simulink model "Pilot"  (R2023b)
settings: Solver=FixedStepAuto  StartTime=0.0  StopTime=inf  FixedStep=sample_time  RelTol=1e-3
model workspace (MAT data in the model file):
  SL_ROS_VariableLengthArrays_MaxSizes.CommonInfo.ArrayTruncateAction = 'EmitWarning'
  SL_ROS_VariableLengthArrays_MaxSizes.MsgTypeMap = containers.Map
  SL_ROS_VariableLengthArrays_MaxSizes.MsgTypeMap.serialization.keys = {'sensor_msgs/Image'}
  SL_ROS_VariableLengthArrays_MaxSizes.MsgTypeMap.serialization.values{1}(1).PropertyName = 'data'
  SL_ROS_VariableLengthArrays_MaxSizes.MsgTypeMap.serialization.values{1}(1).DataType = 'uint8'
  SL_ROS_VariableLengthArrays_MaxSizes.MsgTypeMap.serialization.values{1}(1).MaxLength = 921600
  SL_ROS_VariableLengthArrays_MaxSizes.MsgTypeMap.serialization.values{1}(2).PropertyName = 'encoding'
  SL_ROS_VariableLengthArrays_MaxSizes.MsgTypeMap.serialization.values{1}(2).DataType = 'uint8'
  SL_ROS_VariableLengthArrays_MaxSizes.MsgTypeMap.serialization.values{1}(2).MaxLength = 128
  SL_ROS_VariableLengthArrays_MaxSizes.MsgTypeMap.serialization.uniformity = 0
  SL_ROS_VariableLengthArrays_MaxSizes.MsgTypeMap.serialization.keyType = 'char'
  SL_ROS_VariableLengthArrays_MaxSizes.MsgTypeMap.serialization.valueType = 'any'
  sample_time = 0.1
undefined symbols (not defined in the file or in its folder): duration, vel
libraries: ros2lib x2, vrlib x1, simulink_extras x1
settings Model: Creator=rcasado  LastModifiedBy=Rafa
settings SolverCC: AlgebraicLoopSolver=TrustRegion
settings DataIOCC: ReturnWorkspaceOutputs=off
settings OptimizationCC: EnhancedBackFolding=on  PassReuseOutputArgsAs=Individual arguments  ZeroExternalMemoryAtStartup=off  ZeroInternalMemoryAtStartup=off  MaxStackSize=64  OptimizeBlockOrder=speed  DifferentSizesBufferReuse=on  OptimizationCustomize=off  EfficientTunableParamExpr=on
settings DebuggingCC: ParameterTunabilityLossMsg=error  UnconnectedInputMsg=warning  UnconnectedOutputMsg=warning  UnconnectedLineMsg=warning  BusObjectLabelMismatch=none  PregeneratedLibrarySubsystemCodeDiagnostic=none  ArithmeticOperatorsInVariantConditions=warning
settings HardwareCC: ProdBitPerPointer=32  ProdBitPerSizeT=32  ProdBitPerPtrDiffT=32  ProdLargestAtomicFloat=None  ProdIntDivRoundTo=Undefined  ProdEndianess=Unspecified  ProdWordSize=32  ProdHWDeviceType=Generic->Unspecified (assume 32-bit Generic)
settings ModelReferenceCC: EnableRefExpFcnMdlSchedulingChecks=on
settings SFSimCC: SimUseLocalCustomCode=off  CustomCodeUndefinedFunction=UseInterfaceOnly  SimTargetLang=C++
settings RTWCC: Description=Embedded Coder  SystemTargetFile=ert.tlc  HardwareBoard=Robot Operating System (ROS)  TLCOptions="-aInlineSetEventsForThisBaseRateFcn=TLC_FALSE -aSuppressMultiTaskScheduler=TLC_FALSE  -aRateBasedStepFcn=0"  TemplateMakefile=ert_default_tmf  GenerateReport=on  RTWUseLocalCustomCode=off  Toolchain=Catkin  IncludeHyperlinkInReport=on  LaunchReport=on  TargetLang=C++  GenerateTraceInfo=on  GenerateTraceReport=on  GenerateTraceReportSl=on  GenerateTraceReportSf=on  GenerateTraceReportEml=on  DLArmComputeVersion=19.05
settings CodeAppCC: ForceParamTrailComments=on  IgnoreCustomStorageClasses=off  OperatorAnnotations=on  SimulinkDataObjDesc=on  SFDataObjDesc=on  InsertBlockDesc=on

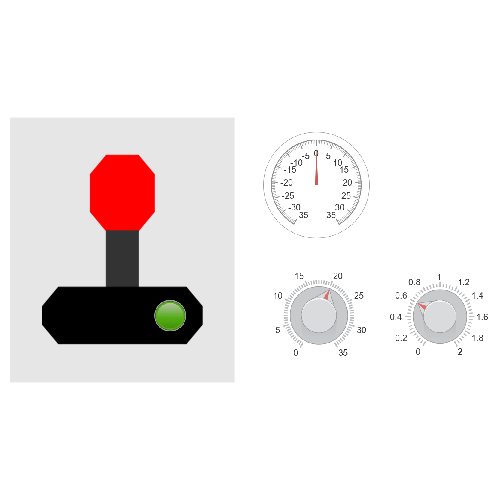
[thumbnail: Simulink's stored preview of the top-level diagram]
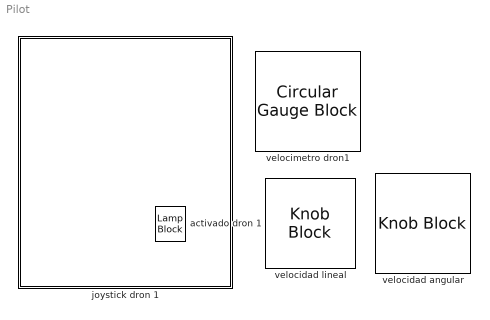
== system Pilot ==
  activado dron 1 : LampBlock  LabelPosition=Hide
  joystick dron 1 : Subsystem
      mask Display:
      | patch([12 -2 -2 12], [12 12 -2 -2], [0.9 0.9 0.9])
      | 
      | % bola roja
      | patch([4 6 7 7 6 4 3 3], [6 6 7 9 10 10 9 7], [1 0 0])
      | 
      | % palo gris
      | patch([4 6 6 4], [3 3 6 6], [0.2 0.2 0.2])
      | 
      | % base negra
      | patch([1 9 10 10 9 1 0 0], [0 0 1 2 3 3 2 1], [0 0 0])
  velocidad angular : KnobBlock  LabelPosition=Hide  ScaleMax=2  TickInterval=0.2
  velocidad lineal : KnobBlock  LabelPosition=Hide  ScaleMax=35  TickInterval=5
  velocimetro dron1 : CircularGaugeBlock  LabelPosition=Hide  ScaleMin=-35  ScaleMax=35  TickInterval=5

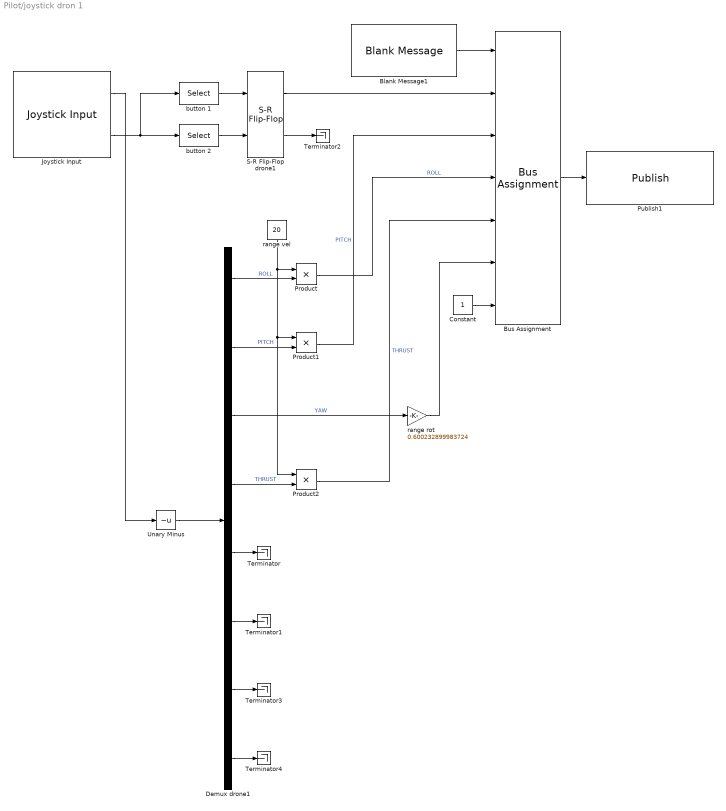
== system Pilot/joystick dron 1 ==
  Blank Message1 : ros2lib/Blank Message  messageClass=Message  entityType=navsim_msgs/RemoteCommand  messageType=navsim_msgs/RemoteCommand  SampleTime=sample_time
  Bus Assignment : BusAssignment  AssignedSignals=on,vel.linear.x,vel.linear.y,vel.linear.z,vel.angular.z,duration.sec
  Constant : Constant  OutDataTypeStr=int32
  Demux drone1 : Demux  Outputs=8
  Joystick Input : vrlib/Joystick Input  joyid=1  adjustports=off  forcefeed=off
  Product : Product
  Product1 : Product
  Product2 : Product
  Publish1 : ros2lib/Publish  topicSource=Select from ROS network  topic=/NavSim/aguila/RemoteCommand  messageType=navsim_msgs/RemoteCommand  QOSHistory=Keep last  QOSDepth=1  QOSReliability=Reliable  QOSDurability=Volatile
  S-R Flip-Flop drone1 : simulink_extras/Flip Flops/S-R Flip-Flop  initial_condition=0
  Terminator{,1..4} (5 alike) : Terminator
  Unary Minus : UnaryMinus
  button 1 : Selector  InputPortWidth=32  IndexOptions=Index vector (dialog)  Indices=[1]  OutputSizes=1
  button 2 : Selector  InputPortWidth=32  IndexOptions=Index vector (dialog)  Indices=[2]  OutputSizes=1
  range rot : Gain  Gain=0.600232899983724
  range vel : Constant  Value=20
  wires:
  Bus Assignment/1 -> Publish1/1
  Blank Message1/1 -> Bus Assignment/1
  Joystick Input/1 -> Unary Minus/1
  Product/1 -> Bus Assignment/4  "ROLL"
  Product1/1 -> Bus Assignment/3  "PITCH"
  Demux drone1/3 -> range rot/1  "YAW"
  Product2/1 -> Bus Assignment/5  "THRUST"
  Joystick Input/2 -> button 2/1, button 1/1
  S-R Flip-Flop drone1/1 -> Bus Assignment/2
  button 2/1 -> S-R Flip-Flop drone1/2
  button 1/1 -> S-R Flip-Flop drone1/1
  S-R Flip-Flop drone1/2 -> Terminator2/1
  Unary Minus/1 -> Demux drone1/1
  Constant/1 -> Bus Assignment/7
  range rot/1 -> Bus Assignment/6
  range vel/1 -> Product/1, Product1/1, Product2/1
  Demux drone1/4 -> Product2/2  "THRUST"
  Demux drone1/2 -> Product1/2  "PITCH"
  Demux drone1/1 -> Product/2  "ROLL"
  Demux drone1/8 -> Terminator4/1
  Demux drone1/7 -> Terminator3/1
  Demux drone1/6 -> Terminator1/1
  Demux drone1/5 -> Terminator/1
